simulink model "Delta"  (Simulink 7.7)
settings: Solver=ode45  StartTime=0.0  StopTime=40.0  RelTol=1e-3
undefined symbols (not defined in the file or in its folder): carriage, Printhead
libraries: mblibv1 x35
settings Model: Creator=Dot Com  LastModifiedBy=Dot Com
settings SimMechanicsCC: VisOnUpdateDiagram=on  VisDuringSimulation=on

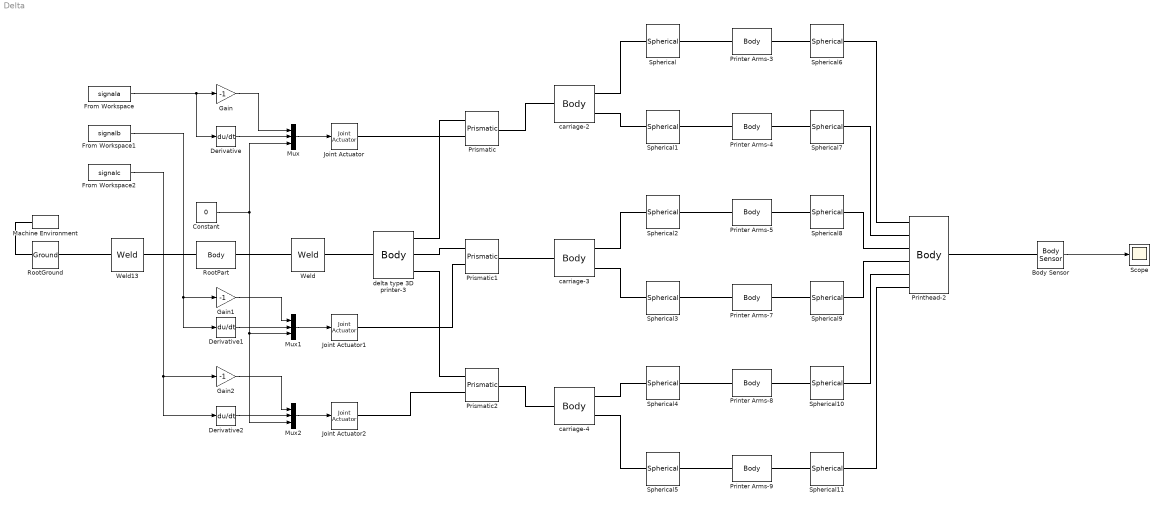
== system Delta ==
  Body Sensor : mblibv1/Sensors &  Actuators/Body Sensor  SystemSampleTime=-1  UpdateFromCAD=off  PhysicalDomain=Mechanical  PortType=blob  Muxed=on  Pose=off  Angle=on  AngleUnits=deg  ArcVelocity=off  ArcVelocityUnits=deg/s  ArcAcceleration=off  ArcAccelerationUnits=deg/s^2  CoordPosition=on  CoordPositionUnits=m  Velocity=off  VelocityUnits=m/s  Acceleration=off  AccelerationUnits=m/s^2  Quaternion=on  QuaternionDT=off  QuaternionDDT=off  QuaternionUnits=off  OutputVector=[1]  ActiveIO=on  Width=3  DialogClass=MechanicalSensorBlock  ReferenceFrame=Absolute (World)
  Constant : Constant  Value=0
  Derivative : Derivative
  Derivative1 : Derivative
  Derivative2 : Derivative
  From Workspace : FromWorkspace  VariableName=signala  SampleTime=0  OutputAfterFinalValue=Holding final value
  From Workspace1 : FromWorkspace  VariableName=signalb  SampleTime=0  OutputAfterFinalValue=Holding final value
  From Workspace2 : FromWorkspace  VariableName=signalc  SampleTime=0  OutputAfterFinalValue=Holding final value
  Gain : Gain  Gain=-1
  Gain1 : Gain  Gain=-1
  Gain2 : Gain  Gain=-1
  Joint Actuator : mblibv1/Sensors &  Actuators/Joint Actuator  SystemSampleTime=-1  UpdateFromCAD=off  PhysicalDomain=Mechanical  PortType=blob  ActuationStyle=Motion  AngleUnits=deg  ArcVelocityUnits=deg/s  ArcAccelerationUnits=deg/s^2  CoordPositionUnits=mm  VelocityUnits=mm/s  AccelerationUnits=mm/s^2  ForceUnits=N  TorqueUnits=N*m  ActiveIO=on  Width=3  DialogClass=MechanicalActuatorBlock  Primitive=P1  ReferenceFrame=Absolute (World)
  Joint Actuator1 : mblibv1/Sensors &  Actuators/Joint Actuator  SystemSampleTime=-1  UpdateFromCAD=off  PhysicalDomain=Mechanical  PortType=blob  ActuationStyle=Motion  AngleUnits=deg  ArcVelocityUnits=deg/s  ArcAccelerationUnits=deg/s^2  CoordPositionUnits=mm  VelocityUnits=mm/s  AccelerationUnits=mm/s^2  ForceUnits=N  TorqueUnits=N*m  ActiveIO=on  Width=3  DialogClass=MechanicalActuatorBlock  Primitive=P1  ReferenceFrame=Absolute (World)
  Joint Actuator2 : mblibv1/Sensors &  Actuators/Joint Actuator  SystemSampleTime=-1  UpdateFromCAD=off  PhysicalDomain=Mechanical  PortType=blob  ActuationStyle=Motion  AngleUnits=deg  ArcVelocityUnits=deg/s  ArcAccelerationUnits=deg/s^2  CoordPositionUnits=mm  VelocityUnits=mm/s  AccelerationUnits=mm/s^2  ForceUnits=N  TorqueUnits=N*m  ActiveIO=on  Width=3  DialogClass=MechanicalActuatorBlock  Primitive=P1  ReferenceFrame=Absolute (World)
  Machine Environment : mblibv1/Bodies/Machine Environment  SystemSampleTime=-1  PortType=env  PhysicalDomain=Mechanical  DialogTemplateClass=MECH.MachineEnvironment  SyncWhenCopied=off  Gravity=[0 -9.81 0]  GravityUnits=m/s^2  GravityAsSignal=off  Dimensionality=Auto-detect  AnalysisType=Forward dynamics  LinearAssemblyTolerance=1e-3  LinearAssemblyToleranceUnits=m  AngularAssemblyTolerance=1e-3  AngularAssemblyToleranceUnits=rad  ConstraintSolverType=Stabilizing  ConstraintRelTolerance=1e-4  ConstraintAbsTolerance=1e-4  UseRobustSingularityHandling=off  RedundancyAnalysisToleranceType=Automatically select tolerance  RedundancyAnalysisTolerance=1e-14  StatePerturbationType=Fixed  PerturbationSize=1e-5  VisualizeMachine=on  BodyVisualizationType=Use model default body geometries  BodyColorSelMode=Use model default  DefaultBodyColor=[1 0 0]
  Mux : Mux  Inputs=3
  Mux1 : Mux  Inputs=3
  Mux2 : Mux  Inputs=3
  Printer Arms-3 : mblibv1/Bodies/Body  PhysicalDomain=mechanical  SubClassName=Unknown  LeftPortType=workingframe  RightPortType=workingframe  LConnTagsString=CS2  RConnTagsString=CS3  UpdateFromCAD=on  PMImportedID=Printer Arms-3  DialogClass=MechanicalBodyBlock  Mass=0.000715383  MassUnits=kg  InertiaUnits=kg*m^2  Inertia=[6.53309e-006,-3.27611e-007,0;-3.27611e-007,1.87881e-008,0;0,0,6.55098e-006]  Shape=Cylinder  ShapeDims=[1 1]  ShapeUnits=m  ShapeUse=false  Density=1  DensityUnits=kg/m^3  DensityUse=false  GraphicsMode=GFXFILE  GraphicsFileName=Delta - Printer Arms-3.STL  BodyColorSelMode=COLORPALETTE  BodyColor=[0.752941;0.752941;0.752941]  AttachedToCS=CS1  CG=Right$CG$[-0.081798 0.287301 0.783358]$WORLD$WORLD$m$[0.856629 -0.438503 0.27185;0.422968 0.898604 0.11666;-0.295441 0.0150491 0.955242]$3x3 Transform$rad$WORLD$false$Printer Arms-3::CG(AUTOGEN)  WorkingFrames=Right$CS1$[0.0652951 0.305355 0.931629]$WORLD$WORLD$m$[0.856629 -0.438503 0.27185;0.422968 0.898604 0.11666;-0.295441 0.0150491 0.955242]$3x3 Transform$rad$WORLD$false$Printer Arms-3::CS1(AUTOGEN)#Left$CS2$[-0.126832 0.392029 0.78339]$WORLD$WORLD$m$[1 0 0;0 1 0;0 0 1]$3x3 Transform$rad$WORLD$true$Printer Arms-3:-:carriage-2::Printer Arms-3(AUTOGEN)#Right$CS3$[-0.0382516 0.186032 0.783333]$WORLD$WORLD$m$[1 0 0;0 1 0;0 0 1]$3x3 Transform$rad$WORLD$true$Printer Arms-3:-:Printhead-2::Printer Arms-3(AUTOGEN)  CGPos=[-0.081798 0.287301 0.783358]  CGRot=[0.856629 -0.438503 0.27185;0.422968 0.898604 0.11666;-0.295441 0.0150491 0.955242]  CS0Pos=[]  CS0Rot=[]  CS1Pos=[0.0652951 0.305355 0.931629]  CS1Rot=[0.856629 -0.438503 0.27185;0.422968 0.898604 0.11666;-0.295441 0.0150491 0.955242]  CS2Pos=[-0.126832 0.392029 0.78339]  CS2Rot=[1 0 0;0 1 0;0 0 1]  CS3Pos=[-0.0382516 0.186032 0.783333]  CS3Rot=[1 0 0;0 1 0;0 0 1]  CS4Pos=[]  CS4Rot=[]  CS5Pos=[]  CS5Rot=[]  CS6Pos=[]  CS6Rot=[]  CS7Pos=[]  CS7Rot=[]  CS8Pos=[]  CS8Rot=[]  CS9Pos=[]  CS9Rot=[]  CS10Pos=[]  CS10Rot=[]  CS11Pos=[]  CS11Rot=[]  CS12Pos=[]  CS12Rot=[]  CS13Pos=[]  CS13Rot=[]  CS14Pos=[]  CS14Rot=[]  CS15Pos=[]  CS15Rot=[]  CS16Pos=[]  CS16Rot=[]  CS17Pos=[]  CS17Rot=[]  CS18Pos=[]  CS18Rot=[]  CS19Pos=[]  CS19Rot=[]  CS20Pos=[]  CS20Rot=[]
  Printer Arms-4 : mblibv1/Bodies/Body  PhysicalDomain=mechanical  SubClassName=Unknown  LeftPortType=workingframe  RightPortType=workingframe  LConnTagsString=CS2  RConnTagsString=CS3  UpdateFromCAD=on  PMImportedID=Printer Arms-4  DialogClass=MechanicalBodyBlock  Mass=0.000715383  MassUnits=kg  InertiaUnits=kg*m^2  Inertia=[6.53309e-006,-3.27611e-007,0;-3.27611e-007,1.87881e-008,0;0,0,6.55098e-006]  Shape=Cylinder  ShapeDims=[1 1]  ShapeUnits=m  ShapeUse=false  Density=1  DensityUnits=kg/m^3  DensityUse=false  GraphicsMode=GFXFILE  GraphicsFileName=Delta - Printer Arms-4.STL  BodyColorSelMode=COLORPALETTE  BodyColor=[0.752941;0.752941;0.752941]  AttachedToCS=CS1  CG=Right$CG$[-0.081798 0.287301 0.744332]$WORLD$WORLD$m$[0.857774 -0.438561 0.268119;0.423387 0.898583 0.115293;-0.29149 0.0146226 0.956462]$3x3 Transform$rad$WORLD$false$Printer Arms-4::CG(AUTOGEN)  WorkingFrames=Right$CS1$[0.0647153 0.305142 0.893201]$WORLD$WORLD$m$[0.857774 -0.438561 0.268119;0.423387 0.898583 0.115293;-0.29149 0.0146226 0.956462]$3x3 Transform$rad$WORLD$false$Printer Arms-4::CS1(AUTOGEN)#Left$CS2$[-0.126832 0.392029 0.744338]$WORLD$WORLD$m$[1 0 0;0 1 0;0 0 1]$3x3 Transform$rad$WORLD$true$Printer Arms-4:-:carriage-2::Printer Arms-4(AUTOGEN)#Right$CS3$[-0.0382516 0.186032 0.744332]$WORLD$WORLD$m$[1 0 0;0 1 0;0 0 1]$3x3 Transform$rad$WORLD$true$Printer Arms-4:-:Printhead-2::Printer Arms-4(AUTOGEN)  CGPos=[-0.081798 0.287301 0.744332]  CGRot=[0.857774 -0.438561 0.268119;0.423387 0.898583 0.115293;-0.29149 0.0146226 0.956462]  CS0Pos=[]  CS0Rot=[]  CS1Pos=[0.0647153 0.305142 0.893201]  CS1Rot=[0.857774 -0.438561 0.268119;0.423387 0.898583 0.115293;-0.29149 0.0146226 0.956462]  CS2Pos=[-0.126832 0.392029 0.744338]  CS2Rot=[1 0 0;0 1 0;0 0 1]  CS3Pos=[-0.0382516 0.186032 0.744332]  CS3Rot=[1 0 0;0 1 0;0 0 1]  CS4Pos=[]  CS4Rot=[]  CS5Pos=[]  CS5Rot=[]  CS6Pos=[]  CS6Rot=[]  CS7Pos=[]  CS7Rot=[]  CS8Pos=[]  CS8Rot=[]  CS9Pos=[]  CS9Rot=[]  CS10Pos=[]  CS10Rot=[]  CS11Pos=[]  CS11Rot=[]  CS12Pos=[]  CS12Rot=[]  CS13Pos=[]  CS13Rot=[]  CS14Pos=[]  CS14Rot=[]  CS15Pos=[]  CS15Rot=[]  CS16Pos=[]  CS16Rot=[]  CS17Pos=[]  CS17Rot=[]  CS18Pos=[]  CS18Rot=[]  CS19Pos=[]  CS19Rot=[]  CS20Pos=[]  CS20Rot=[]
  Printer Arms-5 : mblibv1/Bodies/Body  PhysicalDomain=mechanical  SubClassName=Unknown  LeftPortType=workingframe  RightPortType=workingframe  LConnTagsString=CS2  RConnTagsString=CS3  UpdateFromCAD=on  PMImportedID=Printer Arms-5  DialogClass=MechanicalBodyBlock  Mass=0.000715383  MassUnits=kg  InertiaUnits=kg*m^2  Inertia=[6.53309e-006,-3.27611e-007,0;-3.27611e-007,1.87881e-008,0;0,0,6.55098e-006]  Shape=Cylinder  ShapeDims=[1 1]  ShapeUnits=m  ShapeUse=false  Density=1  DensityUnits=kg/m^3  DensityUse=false  GraphicsMode=GFXFILE  GraphicsFileName=Delta - Printer Arms-5.STL  BodyColorSelMode=COLORPALETTE  BodyColor=[0.752941;0.752941;0.752941]  AttachedToCS=CS1  CG=Right$CG$[0.0520521 0.287301 0.86061]$WORLD$WORLD$m$[0.619598 0.166684 -0.767017;-0.34181 0.936968 -0.0724985;0.706586 0.307094 0.637518]$3x3 Transform$rad$WORLD$false$Printer Arms-5::CG(AUTOGEN)  WorkingFrames=Right$CS1$[-0.0408836 0.200131 1.02708]$WORLD$WORLD$m$[0.619598 0.166684 -0.767017;-0.34181 0.936968 -0.0724985;0.706586 0.307094 0.637518]$3x3 Transform$rad$WORLD$false$Printer Arms-5::CS1(AUTOGEN)#Left$CS2$[0.0745745 0.392029 0.899608]$WORLD$WORLD$m$[1 0 0;0 1 0;0 0 1]$3x3 Transform$rad$WORLD$true$Printer Arms-5:-:carriage-3::Printer Arms-5(AUTOGEN)#Right$CS3$[0.0302789 0.186032 0.822898]$WORLD$WORLD$m$[1 0 0;0 1 0;0 0 1]$3x3 Transform$rad$WORLD$true$Printer Arms-5:-:Printhead-2::Printer Arms-5(AUTOGEN)  CGPos=[0.0520521 0.287301 0.86061]  CGRot=[0.619598 0.166684 -0.767017;-0.34181 0.936968 -0.0724985;0.706586 0.307094 0.637518]  CS0Pos=[]  CS0Rot=[]  CS1Pos=[-0.0408836 0.200131 1.02708]  CS1Rot=[0.619598 0.166684 -0.767017;-0.34181 0.936968 -0.0724985;0.706586 0.307094 0.637518]  CS2Pos=[0.0745745 0.392029 0.899608]  CS2Rot=[1 0 0;0 1 0;0 0 1]  CS3Pos=[0.0302789 0.186032 0.822898]  CS3Rot=[1 0 0;0 1 0;0 0 1]  CS4Pos=[]  CS4Rot=[]  CS5Pos=[]  CS5Rot=[]  CS6Pos=[]  CS6Rot=[]  CS7Pos=[]  CS7Rot=[]  CS8Pos=[]  CS8Rot=[]  CS9Pos=[]  CS9Rot=[]  CS10Pos=[]  CS10Rot=[]  CS11Pos=[]  CS11Rot=[]  CS12Pos=[]  CS12Rot=[]  CS13Pos=[]  CS13Rot=[]  CS14Pos=[]  CS14Rot=[]  CS15Pos=[]  CS15Rot=[]  CS16Pos=[]  CS16Rot=[]  CS17Pos=[]  CS17Rot=[]  CS18Pos=[]  CS18Rot=[]  CS19Pos=[]  CS19Rot=[]  CS20Pos=[]  CS20Rot=[]
  Printer Arms-7 : mblibv1/Bodies/Body  PhysicalDomain=mechanical  SubClassName=Unknown  LeftPortType=workingframe  RightPortType=workingframe  LConnTagsString=CS2  RConnTagsString=CS3  UpdateFromCAD=on  PMImportedID=Printer Arms-7  DialogClass=MechanicalBodyBlock  Mass=0.000715383  MassUnits=kg  InertiaUnits=kg*m^2  Inertia=[6.53309e-006,-3.27611e-007,0;-3.27611e-007,1.87881e-008,0;0,0,6.55098e-006]  Shape=Cylinder  ShapeDims=[1 1]  ShapeUnits=m  ShapeUse=false  Density=1  DensityUnits=kg/m^3  DensityUse=false  GraphicsMode=GFXFILE  GraphicsFileName=Delta - Printer Arms-7.STL  BodyColorSelMode=COLORPALETTE  BodyColor=[0.752941;0.752941;0.752941]  AttachedToCS=CS1  CG=Right$CG$[0.0858496 0.287301 0.841097]$WORLD$WORLD$m$[-0.593901 0.227756 0.771628;0.434444 0.898028 0.0693147;-0.677156 0.376395 -0.632287]$3x3 Transform$rad$WORLD$false$Printer Arms-7::CG(AUTOGEN)  WorkingFrames=Right$CS1$[0.163779 0.297714 0.646765]$WORLD$WORLD$m$[-0.593901 0.227756 0.771628;0.434444 0.898028 0.0693147;-0.677156 0.376395 -0.632287]$3x3 Transform$rad$WORLD$false$Printer Arms-7::CS1(AUTOGEN)#Left$CS2$[0.108395 0.392029 0.880082]$WORLD$WORLD$m$[1 0 0;0 1 0;0 0 1]$3x3 Transform$rad$WORLD$true$Printer Arms-7:-:carriage-3::Printer Arms-7(AUTOGEN)#Right$CS3$[0.0640546 0.186032 0.803398]$WORLD$WORLD$m$[1 0 0;0 1 0;0 0 1]$3x3 Transform$rad$WORLD$true$Printer Arms-7:-:Printhead-2::Printer Arms-7(AUTOGEN)  CGPos=[0.0858496 0.287301 0.841097]  CGRot=[-0.593901 0.227756 0.771628;0.434444 0.898028 0.0693147;-0.677156 0.376395 -0.632287]  CS0Pos=[]  CS0Rot=[]  CS1Pos=[0.163779 0.297714 0.646765]  CS1Rot=[-0.593901 0.227756 0.771628;0.434444 0.898028 0.0693147;-0.677156 0.376395 -0.632287]  CS2Pos=[0.108395 0.392029 0.880082]  CS2Rot=[1 0 0;0 1 0;0 0 1]  CS3Pos=[0.0640546 0.186032 0.803398]  CS3Rot=[1 0 0;0 1 0;0 0 1]  CS4Pos=[]  CS4Rot=[]  CS5Pos=[]  CS5Rot=[]  CS6Pos=[]  CS6Rot=[]  CS7Pos=[]  CS7Rot=[]  CS8Pos=[]  CS8Rot=[]  CS9Pos=[]  CS9Rot=[]  CS10Pos=[]  CS10Rot=[]  CS11Pos=[]  CS11Rot=[]  CS12Pos=[]  CS12Rot=[]  CS13Pos=[]  CS13Rot=[]  CS14Pos=[]  CS14Rot=[]  CS15Pos=[]  CS15Rot=[]  CS16Pos=[]  CS16Rot=[]  CS17Pos=[]  CS17Rot=[]  CS18Pos=[]  CS18Rot=[]  CS19Pos=[]  CS19Rot=[]  CS20Pos=[]  CS20Rot=[]
  Printer Arms-8 : mblibv1/Bodies/Body  PhysicalDomain=mechanical  SubClassName=Unknown  LeftPortType=workingframe  RightPortType=workingframe  LConnTagsString=CS2  RConnTagsString=CS3  UpdateFromCAD=on  PMImportedID=Printer Arms-8  DialogClass=MechanicalBodyBlock  Mass=0.000715383  MassUnits=kg  InertiaUnits=kg*m^2  Inertia=[6.53309e-006,-3.27611e-007,0;-3.27611e-007,1.87881e-008,0;0,0,6.55098e-006]  Shape=Cylinder  ShapeDims=[1 1]  ShapeUnits=m  ShapeUse=false  Density=1  DensityUnits=kg/m^3  DensityUse=false  GraphicsMode=GFXFILE  GraphicsFileName=Delta - Printer Arms-8.STL  BodyColorSelMode=COLORPALETTE  BodyColor=[0.752941;0.752941;0.752941]  AttachedToCS=CS1  CG=Right$CG$[0.0520296 0.287301 0.667041]$WORLD$WORLD$m$[-0.253842 0.210301 -0.944107;0.431532 0.898174 0.0840436;0.865647 -0.386079 -0.318746]$3x3 Transform$rad$WORLD$false$Printer Arms-8::CG(AUTOGEN)  WorkingFrames=Right$CS1$[-0.153917 0.300151 0.704021]$WORLD$WORLD$m$[-0.253842 0.210301 -0.944107;0.431532 0.898174 0.0840436;0.865647 -0.386079 -0.318746]$3x3 Transform$rad$WORLD$false$Printer Arms-8::CS1(AUTOGEN)#Left$CS2$[0.0745185 0.392029 0.628024]$WORLD$WORLD$m$[1 0 0;0 1 0;0 0 1]$3x3 Transform$rad$WORLD$true$Printer Arms-8:-:carriage-4::Printer Arms-8(AUTOGEN)#Right$CS3$[0.0302782 0.186032 0.704766]$WORLD$WORLD$m$[1 0 0;0 1 0;0 0 1]$3x3 Transform$rad$WORLD$true$Printer Arms-8:-:Printhead-2::Printer Arms-8(AUTOGEN)  CGPos=[0.0520296 0.287301 0.667041]  CGRot=[-0.253842 0.210301 -0.944107;0.431532 0.898174 0.0840436;0.865647 -0.386079 -0.318746]  CS0Pos=[]  CS0Rot=[]  CS1Pos=[-0.153917 0.300151 0.704021]  CS1Rot=[-0.253842 0.210301 -0.944107;0.431532 0.898174 0.0840436;0.865647 -0.386079 -0.318746]  CS2Pos=[0.0745185 0.392029 0.628024]  CS2Rot=[1 0 0;0 1 0;0 0 1]  CS3Pos=[0.0302782 0.186032 0.704766]  CS3Rot=[1 0 0;0 1 0;0 0 1]  CS4Pos=[]  CS4Rot=[]  CS5Pos=[]  CS5Rot=[]  CS6Pos=[]  CS6Rot=[]  CS7Pos=[]  CS7Rot=[]  CS8Pos=[]  CS8Rot=[]  CS9Pos=[]  CS9Rot=[]  CS10Pos=[]  CS10Rot=[]  CS11Pos=[]  CS11Rot=[]  CS12Pos=[]  CS12Rot=[]  CS13Pos=[]  CS13Rot=[]  CS14Pos=[]  CS14Rot=[]  CS15Pos=[]  CS15Rot=[]  CS16Pos=[]  CS16Rot=[]  CS17Pos=[]  CS17Rot=[]  CS18Pos=[]  CS18Rot=[]  CS19Pos=[]  CS19Rot=[]  CS20Pos=[]  CS20Rot=[]
  Printer Arms-9 : mblibv1/Bodies/Body  PhysicalDomain=mechanical  SubClassName=Unknown  LeftPortType=workingframe  RightPortType=workingframe  LConnTagsString=CS2  RConnTagsString=CS3  UpdateFromCAD=on  PMImportedID=Printer Arms-9  DialogClass=MechanicalBodyBlock  Mass=0.000715383  MassUnits=kg  InertiaUnits=kg*m^2  Inertia=[6.53309e-006,-3.27611e-007,0;-3.27611e-007,1.87881e-008,0;0,0,6.55098e-006]  Shape=Cylinder  ShapeDims=[1 1]  ShapeUnits=m  ShapeUse=false  Density=1  DensityUnits=kg/m^3  DensityUse=false  GraphicsMode=GFXFILE  GraphicsFileName=Delta - Printer Arms-9.STL  BodyColorSelMode=COLORPALETTE  BodyColor=[0.752941;0.752941;0.752941]  AttachedToCS=CS1  CG=Right$CG$[0.0858271 0.287301 0.686554]$WORLD$WORLD$m$[-0.257215 0.210668 -0.943111;0.431786 0.898161 0.0828664;0.864524 -0.385908 -0.321984]$3x3 Transform$rad$WORLD$false$Printer Arms-9::CG(AUTOGEN)  WorkingFrames=Right$CS1$[-0.120256 0.299959 0.72283]$WORLD$WORLD$m$[-0.257215 0.210668 -0.943111;0.431786 0.898161 0.0828664;0.864524 -0.385908 -0.321984]$3x3 Transform$rad$WORLD$false$Printer Arms-9::CS1(AUTOGEN)#Left$CS2$[0.108339 0.392029 0.64755]$WORLD$WORLD$m$[1 0 0;0 1 0;0 0 1]$3x3 Transform$rad$WORLD$true$Printer Arms-9:-:carriage-4::Printer Arms-9(AUTOGEN)#Right$CS3$[0.0640539 0.186032 0.724266]$WORLD$WORLD$m$[1 0 0;0 1 0;0 0 1]$3x3 Transform$rad$WORLD$true$Printer Arms-9:-:Printhead-2::Printer Arms-9(AUTOGEN)  CGPos=[0.0858271 0.287301 0.686554]  CGRot=[-0.257215 0.210668 -0.943111;0.431786 0.898161 0.0828664;0.864524 -0.385908 -0.321984]  CS0Pos=[]  CS0Rot=[]  CS1Pos=[-0.120256 0.299959 0.72283]  CS1Rot=[-0.257215 0.210668 -0.943111;0.431786 0.898161 0.0828664;0.864524 -0.385908 -0.321984]  CS2Pos=[0.108339 0.392029 0.64755]  CS2Rot=[1 0 0;0 1 0;0 0 1]  CS3Pos=[0.0640539 0.186032 0.724266]  CS3Rot=[1 0 0;0 1 0;0 0 1]  CS4Pos=[]  CS4Rot=[]  CS5Pos=[]  CS5Rot=[]  CS6Pos=[]  CS6Rot=[]  CS7Pos=[]  CS7Rot=[]  CS8Pos=[]  CS8Rot=[]  CS9Pos=[]  CS9Rot=[]  CS10Pos=[]  CS10Rot=[]  CS11Pos=[]  CS11Rot=[]  CS12Pos=[]  CS12Rot=[]  CS13Pos=[]  CS13Rot=[]  CS14Pos=[]  CS14Rot=[]  CS15Pos=[]  CS15Rot=[]  CS16Pos=[]  CS16Rot=[]  CS17Pos=[]  CS17Rot=[]  CS18Pos=[]  CS18Rot=[]  CS19Pos=[]  CS19Rot=[]  CS20Pos=[]  CS20Rot=[]
  Printhead-2 : mblibv1/Bodies/Body  PhysicalDomain=mechanical  SubClassName=Unknown  LeftPortType=workingframe  RightPortType=workingframe  LConnTagsString=CS2|CS3|CS4|CS5|CS6|CS7  RConnTagsString=CS1  UpdateFromCAD=on  PMImportedID=Printhead-2  DialogClass=MechanicalBodyBlock  Mass=0.132596  MassUnits=kg  InertiaUnits=kg*m^2  Inertia=[0.000117863,0,0;0,0.000230731,0;0,0,0.000117863]  Shape=Cylinder  ShapeDims=[1 1]  ShapeUnits=m  ShapeUse=false  Density=1  DensityUnits=kg/m^3  DensityUse=false  GraphicsMode=GFXFILE  GraphicsFileName=Delta - Printhead-2.STL  BodyColorSelMode=COLORPALETTE  BodyColor=[0.75294 0.75294 0.75294]  AttachedToCS=CS1  CG=Right$CG$[0.0186937 0.182574 0.763832]$WORLD$WORLD$m$[-3.8521e-007 0 -1;-1.23652e-012 1 0;1 1.23652e-012 -3.8521e-007]$3x3 Transform$rad$WORLD$false$Printhead-2::CG(AUTOGEN)  WorkingFrames=Right$CS1$[0.146711 0.19172 0.763551]$WORLD$WORLD$m$[-3.8521e-007 0 -1;-1.23652e-012 1 0;1 1.23652e-012 -3.8521e-007]$3x3 Transform$rad$WORLD$true$Printhead-2::CS1(AUTOGEN)#Left$CS2$[-0.0382516 0.186032 0.783333]$WORLD$WORLD$m$[1 0 0;0 1 0;0 0 1]$3x3 Transform$rad$WORLD$true$Printer Arms-3:-:Printhead-2::Printhead-2(AUTOGEN)#Left$CS3$[-0.0382516 0.186032 0.744332]$WORLD$WORLD$m$[1 0 0;0 1 0;0 0 1]$3x3 Transform$rad$WORLD$true$Printer Arms-4:-:Printhead-2::Printhead-2(AUTOGEN)#Left$CS4$[0.0302789 0.186032 0.822898]$WORLD$WORLD$m$[1 0 0;0 1 0;0 0 1]$3x3 Transform$rad$WORLD$true$Printer Arms-5:-:Printhead-2::Printhead-2(AUTOGEN)#Left$CS5$[0.0640546 0.186032 0.803398]$WORLD$WORLD$m$[1 0 0;0 1 0;0 0 1]$3x3 Transform$rad$WORLD$true$Printer Arms-7:-:Printhead-2::Printhead-2(AUTOGEN)#Left$CS6$[0.0302782 0.186032 0.704766]$WORLD$WORLD$m$[1 0 0;0 1 0;0 0 1]$3x3 Transform$rad$WORLD$true$Printer Arms-8:-:Printhead-2::Printhead-2(AUTOGEN)#Left$CS7$[0.0640539 0.186032 0.724266]$WORLD$WORLD$m$[1 0 0;0 1 0;0 0 1]$3x3 Transform$rad$WORLD$true$Printer Arms-9:-:Printhead-2::Printhead-2(AUTOGEN)  CGPos=[0.0186937 0.182574 0.763832]  CGRot=[-3.8521e-007 0 -1;-1.23652e-012 1 0;1 1.23652e-012 -3.8521e-007]  CS0Pos=[]  CS0Rot=[]  CS1Pos=[0.146711 0.19172 0.763551]  CS1Rot=[-3.8521e-007 0 -1;-1.23652e-012 1 0;1 1.23652e-012 -3.8521e-007]  CS2Pos=[-0.0382516 0.186032 0.783333]  CS2Rot=[1 0 0;0 1 0;0 0 1]  CS3Pos=[-0.0382516 0.186032 0.744332]  CS3Rot=[1 0 0;0 1 0;0 0 1]  CS4Pos=[0.0302789 0.186032 0.822898]  CS4Rot=[1 0 0;0 1 0;0 0 1]  CS5Pos=[0.0640546 0.186032 0.803398]  CS5Rot=[1 0 0;0 1 0;0 0 1]  CS6Pos=[0.0302782 0.186032 0.704766]  CS6Rot=[1 0 0;0 1 0;0 0 1]  CS7Pos=[0.0640539 0.186032 0.724266]  CS7Rot=[1 0 0;0 1 0;0 0 1]  CS8Pos=[]  CS8Rot=[]  CS9Pos=[]  CS9Rot=[]  CS10Pos=[]  CS10Rot=[]  CS11Pos=[]  CS11Rot=[]  CS12Pos=[]  CS12Rot=[]  CS13Pos=[]  CS13Rot=[]  CS14Pos=[]  CS14Rot=[]  CS15Pos=[]  CS15Rot=[]  CS16Pos=[]  CS16Rot=[]  CS17Pos=[]  CS17Rot=[]  CS18Pos=[]  CS18Rot=[]  CS19Pos=[]  CS19Rot=[]  CS20Pos=[]  CS20Rot=[]
  Prismatic : mblibv1/Joints/Prismatic  PhysicalDomain=mechanical  SubClassName=Unknown  LeftPortType=blob  RightPortType=blob  LConnTagsString=__newl0|SA1  RConnTagsString=__newr0  UpdateFromCAD=on  PMImportedID=carriage-2:-:delta type 3D printer-3  NumSAPorts=1  CutJoint=off  MarkAsCut=off  Primitives=prismatic  PrimitiveProps=P1$World$[0,1,0]$prismatic  DialogClass=JointBlock  P1Axis=[0,1,0]
  Prismatic1 : mblibv1/Joints/Prismatic  PhysicalDomain=mechanical  SubClassName=Unknown  LeftPortType=blob  RightPortType=blob  LConnTagsString=__newl0|SA1  RConnTagsString=__newr0  UpdateFromCAD=on  PMImportedID=carriage-3:-:delta type 3D printer-3  NumSAPorts=1  CutJoint=off  MarkAsCut=off  Primitives=prismatic  PrimitiveProps=P1$World$[0,1,0]$prismatic  DialogClass=JointBlock  P1Axis=[0,1,0]
  Prismatic2 : mblibv1/Joints/Prismatic  PhysicalDomain=mechanical  SubClassName=Unknown  LeftPortType=blob  RightPortType=blob  LConnTagsString=__newl0|SA1  RConnTagsString=__newr0  UpdateFromCAD=on  PMImportedID=carriage-4:-:delta type 3D printer-3  NumSAPorts=1  CutJoint=off  MarkAsCut=off  Primitives=prismatic  PrimitiveProps=P1$World$[0,1,0]$prismatic  DialogClass=JointBlock  P1Axis=[0,1,0]
  RootGround : mblibv1/Bodies/Ground  SystemSampleTime=-1  UpdateFromCAD=on  PMImportedID=RootGround  LeftPortType=env  RightPortType=workingframe  PhysicalDomain=Mechanical  DialogClass=GroundBlock  CoordPosition=[0.0186634,0.0298068,0.763791]  CoordPositionUnits=m  StateVectorMgrId=1  MachineId=[2 0]  ShowEnvPort=on
  RootPart : mblibv1/Bodies/Body  PhysicalDomain=mechanical  SubClassName=Unknown  LeftPortType=workingframe  RightPortType=workingframe  LConnTagsString=CS3  RConnTagsString=CS2  UpdateFromCAD=on  PMImportedID=Delta/RootPart  DialogClass=MechanicalBodyBlock  Mass=0  MassUnits=kg  InertiaUnits=kg*m^2  Inertia=[0,0,0;0,0,0;0,0,0]  Shape=Cylinder  ShapeDims=[1 1]  ShapeUnits=m  ShapeUse=false  Density=1  DensityUnits=kg/m^3  DensityUse=false  GraphicsMode=MACHINE_DEFAULT  BodyColorSelMode=MACHINE_DEFAULT  BodyColor=[1;0;0]  AttachedToCS=CS1  CG=Right$CG$[0.0186634 0.0298068 0.763791]$WORLD$WORLD$m$[1 0 0;0 1 0;0 0 1]$3x3 Transform$rad$WORLD$false$Delta/RootPart::CG(AUTOGEN)  WorkingFrames=Right$CS1$[0 0 0]$WORLD$WORLD$m$[1 0 0;0 1 0;0 0 1]$3x3 Transform$rad$WORLD$false$Delta/RootPart::CS1(AUTOGEN)#Right$CS2$[0.0186587 -0.0166149 0.763785]$WORLD$WORLD$m$[1 0 0;0 1 0;0 0 1]$3x3 Transform$rad$WORLD$true$Delta/RootPart:-:delta type 3D printer-3::Delta/RootPart(AUTOGEN)#Left$CS3$[0.0186634 0.0298068 0.763791]$WORLD$WORLD$m$[1 0 0;0 1 0;0 0 1]$3x3 Transform$rad$WORLD$true$Delta/RootPart:-:RootGround::Delta/RootPart(AUTOGEN)  CGPos=[0.0186634 0.0298068 0.763791]  CGRot=[1 0 0;0 1 0;0 0 1]  CS0Pos=[]  CS0Rot=[]  CS1Pos=[0 0 0]  CS1Rot=[1 0 0;0 1 0;0 0 1]  CS2Pos=[0.0186587 -0.0166149 0.763785]  CS2Rot=[1 0 0;0 1 0;0 0 1]  CS3Pos=[0.0186634 0.0298068 0.763791]  CS3Rot=[1 0 0;0 1 0;0 0 1]  CS4Pos=[]  CS4Rot=[]  CS5Pos=[]  CS5Rot=[]  CS6Pos=[]  CS6Rot=[]  CS7Pos=[]  CS7Rot=[]  CS8Pos=[]  CS8Rot=[]  CS9Pos=[]  CS9Rot=[]  CS10Pos=[]  CS10Rot=[]  CS11Pos=[]  CS11Rot=[]  CS12Pos=[]  CS12Rot=[]  CS13Pos=[]  CS13Rot=[]  CS14Pos=[]  CS14Rot=[]  CS15Pos=[]  CS15Rot=[]  CS16Pos=[]  CS16Rot=[]  CS17Pos=[]  CS17Rot=[]  CS18Pos=[]  CS18Rot=[]  CS19Pos=[]  CS19Rot=[]  CS20Pos=[]  CS20Rot=[]
  Scope : Scope
  Spherical{,1..11} (12 alike) : mblibv1/Joints/Spherical  PhysicalDomain=mechanical  SubClassName=Unknown  LeftPortType=blob  RightPortType=blob  LConnTagsString=__newl0  RConnTagsString=__newr0  UpdateFromCAD=off  NumSAPorts=0  CutJoint=off  MarkAsCut=off  Primitives=spherical  PrimitiveProps=S$WORLD$[0 0 0]$spherical  DialogClass=JointBlock  SAxis=[0 0 0]
  Weld : mblibv1/Joints/Weld  PhysicalDomain=mechanical  SubClassName=Unknown  LeftPortType=blob  RightPortType=blob  LConnTagsString=__newl0  RConnTagsString=__newr0  UpdateFromCAD=on  PMImportedID=Delta/RootPart:-:delta type 3D printer-3  NumSAPorts=0  CutJoint=off  MarkAsCut=off  Primitives=weld  PrimitiveProps=W$WORLD$[0.57735,0.57735,0.57735]$weld  DialogClass=JointBlock  WAxis=[0.57735,0.57735,0.57735]
  Weld13 : mblibv1/Joints/Weld  PhysicalDomain=mechanical  SubClassName=Unknown  LeftPortType=blob  RightPortType=blob  LConnTagsString=__newl0  RConnTagsString=__newr0  UpdateFromCAD=on  PMImportedID=Delta/RootPart:-:RootGround  NumSAPorts=0  CutJoint=off  MarkAsCut=off  Primitives=weld  PrimitiveProps=W$WORLD$[0.57735,0.57735,0.57735]$weld  DialogClass=JointBlock  WAxis=[0.57735,0.57735,0.57735]
  carriage-2 : mblibv1/Bodies/Body  PhysicalDomain=mechanical  SubClassName=Unknown  LeftPortType=workingframe  RightPortType=workingframe  LConnTagsString=CS2  RConnTagsString=CS3|CS4  UpdateFromCAD=on  PMImportedID=carriage-2  DialogClass=MechanicalBodyBlock  Mass=0.119531  MassUnits=kg  InertiaUnits=kg*m^2  Inertia=[8.71516e-005,1.3952e-008,-7.11667e-010;1.3952e-008,0.000105618,4.08463e-013;-7.11667e-010,4.08463e-013,5.02939e-005]  Shape=Cylinder  ShapeDims=[1 1]  ShapeUnits=m  ShapeUse=false  Density=1  DensityUnits=kg/m^3  DensityUse=false  GraphicsMode=GFXFILE  GraphicsFileName=Delta - carriage-2.STL  BodyColorSelMode=COLORPALETTE  BodyColor=[0.752941;0.752941;0.752941]  AttachedToCS=CS1  CG=Right$CG$[-0.146483 0.392017 0.763832]$WORLD$WORLD$m$[-1 0 0;0 1 0;0 0 -1]$3x3 Transform$rad$WORLD$false$carriage-2::CG(AUTOGEN)  WorkingFrames=Right$CS1$[-0.157413 0.388666 0.853832]$WORLD$WORLD$m$[-1 0 0;0 1 0;0 0 -1]$3x3 Transform$rad$WORLD$false$carriage-2::CS1(AUTOGEN)#Left$CS2$[-0.156832 0.412029 0.733832]$WORLD$WORLD$m$[1 0 0;0 1 0;0 0 1]$3x3 Transform$rad$WORLD$true$carriage-2:-:delta type 3D printer-3::carriage-2(AUTOGEN)#Right$CS3$[-0.126832 0.392029 0.78339]$WORLD$WORLD$m$[1 0 0;0 1 0;0 0 1]$3x3 Transform$rad$WORLD$true$Printer Arms-3:-:carriage-2::carriage-2(AUTOGEN)#Right$CS4$[-0.126832 0.392029 0.744338]$WORLD$WORLD$m$[1 0 0;0 1 0;0 0 1]$3x3 Transform$rad$WORLD$true$Printer Arms-4:-:carriage-2::carriage-2(AUTOGEN)  CGPos=[-0.146483 0.392017 0.763832]  CGRot=[-1 0 0;0 1 0;0 0 -1]  CS0Pos=[]  CS0Rot=[]  CS1Pos=[-0.157413 0.388666 0.853832]  CS1Rot=[-1 0 0;0 1 0;0 0 -1]  CS2Pos=[-0.156832 0.412029 0.733832]  CS2Rot=[1 0 0;0 1 0;0 0 1]  CS3Pos=[-0.126832 0.392029 0.78339]  CS3Rot=[1 0 0;0 1 0;0 0 1]  CS4Pos=[-0.126832 0.392029 0.744338]  CS4Rot=[1 0 0;0 1 0;0 0 1]  CS5Pos=[]  CS5Rot=[]  CS6Pos=[]  CS6Rot=[]  CS7Pos=[]  CS7Rot=[]  CS8Pos=[]  CS8Rot=[]  CS9Pos=[]  CS9Rot=[]  CS10Pos=[]  CS10Rot=[]  CS11Pos=[]  CS11Rot=[]  CS12Pos=[]  CS12Rot=[]  CS13Pos=[]  CS13Rot=[]  CS14Pos=[]  CS14Rot=[]  CS15Pos=[]  CS15Rot=[]  CS16Pos=[]  CS16Rot=[]  CS17Pos=[]  CS17Rot=[]  CS18Pos=[]  CS18Rot=[]  CS19Pos=[]  CS19Rot=[]  CS20Pos=[]  CS20Rot=[]
  carriage-3 : mblibv1/Bodies/Body  PhysicalDomain=mechanical  SubClassName=Unknown  LeftPortType=workingframe  RightPortType=workingframe  LConnTagsString=CS2  RConnTagsString=CS3|CS4  UpdateFromCAD=on  PMImportedID=carriage-3  DialogClass=MechanicalBodyBlock  Mass=0.119531  MassUnits=kg  InertiaUnits=kg*m^2  Inertia=[8.71516e-005,1.3952e-008,-7.11667e-010;1.3952e-008,0.000105618,4.08463e-013;-7.11667e-010,4.08463e-013,5.02939e-005]  Shape=Cylinder  ShapeDims=[1 1]  ShapeUnits=m  ShapeUse=false  Density=1  DensityUnits=kg/m^3  DensityUse=false  GraphicsMode=GFXFILE  GraphicsFileName=Delta - carriage-3.STL  BodyColorSelMode=COLORPALETTE  BodyColor=[0.752941;0.752941;0.752941]  AttachedToCS=CS1  CG=Right$CG$[0.101282 0.392017 0.906879]$WORLD$WORLD$m$[0.5 0 -0.866025;0 1 0;0.866025 0 0.5]$3x3 Transform$rad$WORLD$false$carriage-3::CG(AUTOGEN)  WorkingFrames=Right$CS1$[0.184689 0.388666 0.871345]$WORLD$WORLD$m$[0.5 0 -0.866025;0 1 0;0.866025 0 0.5]$3x3 Transform$rad$WORLD$false$carriage-3::CS1(AUTOGEN)#Left$CS2$[0.0804758 0.412029 0.930842]$WORLD$WORLD$m$[1 0 0;0 1 0;0 0 1]$3x3 Transform$rad$WORLD$true$carriage-3:-:delta type 3D printer-3::carriage-3(AUTOGEN)#Right$CS3$[0.0745745 0.392029 0.899608]$WORLD$WORLD$m$[1 0 0;0 1 0;0 0 1]$3x3 Transform$rad$WORLD$true$Printer Arms-5:-:carriage-3::carriage-3(AUTOGEN)#Right$CS4$[0.108395 0.392029 0.880082]$WORLD$WORLD$m$[1 0 0;0 1 0;0 0 1]$3x3 Transform$rad$WORLD$true$Printer Arms-7:-:carriage-3::carriage-3(AUTOGEN)  CGPos=[0.101282 0.392017 0.906879]  CGRot=[0.5 0 -0.866025;0 1 0;0.866025 0 0.5]  CS0Pos=[]  CS0Rot=[]  CS1Pos=[0.184689 0.388666 0.871345]  CS1Rot=[0.5 0 -0.866025;0 1 0;0.866025 0 0.5]  CS2Pos=[0.0804758 0.412029 0.930842]  CS2Rot=[1 0 0;0 1 0;0 0 1]  CS3Pos=[0.0745745 0.392029 0.899608]  CS3Rot=[1 0 0;0 1 0;0 0 1]  CS4Pos=[0.108395 0.392029 0.880082]  CS4Rot=[1 0 0;0 1 0;0 0 1]  CS5Pos=[]  CS5Rot=[]  CS6Pos=[]  CS6Rot=[]  CS7Pos=[]  CS7Rot=[]  CS8Pos=[]  CS8Rot=[]  CS9Pos=[]  CS9Rot=[]  CS10Pos=[]  CS10Rot=[]  CS11Pos=[]  CS11Rot=[]  CS12Pos=[]  CS12Rot=[]  CS13Pos=[]  CS13Rot=[]  CS14Pos=[]  CS14Rot=[]  CS15Pos=[]  CS15Rot=[]  CS16Pos=[]  CS16Rot=[]  CS17Pos=[]  CS17Rot=[]  CS18Pos=[]  CS18Rot=[]  CS19Pos=[]  CS19Rot=[]  CS20Pos=[]  CS20Rot=[]
  carriage-4 : mblibv1/Bodies/Body  PhysicalDomain=mechanical  SubClassName=Unknown  LeftPortType=workingframe  RightPortType=workingframe  LConnTagsString=CS2  RConnTagsString=CS3|CS4  UpdateFromCAD=on  PMImportedID=carriage-4  DialogClass=MechanicalBodyBlock  Mass=0.119531  MassUnits=kg  InertiaUnits=kg*m^2  Inertia=[8.71516e-005,1.3952e-008,-7.11667e-010;1.3952e-008,0.000105618,4.08463e-013;-7.11667e-010,4.08463e-013,5.02939e-005]  Shape=Cylinder  ShapeDims=[1 1]  ShapeUnits=m  ShapeUse=false  Density=1  DensityUnits=kg/m^3  DensityUse=false  GraphicsMode=GFXFILE  GraphicsFileName=Delta - carriage-4.STL  BodyColorSelMode=COLORPALETTE  BodyColor=[0.752941;0.752941;0.752941]  AttachedToCS=CS1  CG=Right$CG$[0.101282 0.392017 0.620785]$WORLD$WORLD$m$[0.5 0 0.866025;0 1 0;-0.866025 0 0.5]$3x3 Transform$rad$WORLD$false$carriage-4::CG(AUTOGEN)  WorkingFrames=Right$CS1$[0.0288049 0.388666 0.566319]$WORLD$WORLD$m$[0.5 0 0.866025;0 1 0;-0.866025 0 0.5]$3x3 Transform$rad$WORLD$false$carriage-4::CS1(AUTOGEN)#Left$CS2$[0.0804758 0.412029 0.596822]$WORLD$WORLD$m$[1 0 0;0 1 0;0 0 1]$3x3 Transform$rad$WORLD$true$carriage-4:-:delta type 3D printer-3::carriage-4(AUTOGEN)#Right$CS3$[0.0745185 0.392029 0.628024]$WORLD$WORLD$m$[1 0 0;0 1 0;0 0 1]$3x3 Transform$rad$WORLD$true$Printer Arms-8:-:carriage-4::carriage-4(AUTOGEN)#Right$CS4$[0.108339 0.392029 0.64755]$WORLD$WORLD$m$[1 0 0;0 1 0;0 0 1]$3x3 Transform$rad$WORLD$true$Printer Arms-9:-:carriage-4::carriage-4(AUTOGEN)  CGPos=[0.101282 0.392017 0.620785]  CGRot=[0.5 0 0.866025;0 1 0;-0.866025 0 0.5]  CS0Pos=[]  CS0Rot=[]  CS1Pos=[0.0288049 0.388666 0.566319]  CS1Rot=[0.5 0 0.866025;0 1 0;-0.866025 0 0.5]  CS2Pos=[0.0804758 0.412029 0.596822]  CS2Rot=[1 0 0;0 1 0;0 0 1]  CS3Pos=[0.0745185 0.392029 0.628024]  CS3Rot=[1 0 0;0 1 0;0 0 1]  CS4Pos=[0.108339 0.392029 0.64755]  CS4Rot=[1 0 0;0 1 0;0 0 1]  CS5Pos=[]  CS5Rot=[]  CS6Pos=[]  CS6Rot=[]  CS7Pos=[]  CS7Rot=[]  CS8Pos=[]  CS8Rot=[]  CS9Pos=[]  CS9Rot=[]  CS10Pos=[]  CS10Rot=[]  CS11Pos=[]  CS11Rot=[]  CS12Pos=[]  CS12Rot=[]  CS13Pos=[]  CS13Rot=[]  CS14Pos=[]  CS14Rot=[]  CS15Pos=[]  CS15Rot=[]  CS16Pos=[]  CS16Rot=[]  CS17Pos=[]  CS17Rot=[]  CS18Pos=[]  CS18Rot=[]  CS19Pos=[]  CS19Rot=[]  CS20Pos=[]  CS20Rot=[]
  delta type 3D printer-3 : mblibv1/Bodies/Body  PhysicalDomain=mechanical  SubClassName=Unknown  LeftPortType=workingframe  RightPortType=workingframe  LConnTagsString=CS2  RConnTagsString=CS3|CS4|CS5  UpdateFromCAD=on  PMImportedID=delta type 3D printer-3  DialogClass=MechanicalBodyBlock  Mass=3.25813  MassUnits=kg  InertiaUnits=kg*m^2  Inertia=[0.36389,-2.65999e-006,3.41661e-005;-2.65999e-006,0.36387,2.64566e-005;3.41661e-005,2.64566e-005,0.0593532]  Shape=Cylinder  ShapeDims=[1 1]  ShapeUnits=m  ShapeUse=false  Density=1  DensityUnits=kg/m^3  DensityUse=false  GraphicsMode=GFXFILE  GraphicsFileName=Delta - delta type 3D printer-3.STL  BodyColorSelMode=COLORPALETTE  BodyColor=[0.752941;0.752941;0.752941]  AttachedToCS=CS1  CG=Right$CG$[0.0186587 -0.0166149 0.763785]$WORLD$WORLD$m$[0 -1 0;0 0 1;-1 0 0]$3x3 Transform$rad$WORLD$false$delta type 3D printer-3::CG(AUTOGEN)  WorkingFrames=Right$CS1$[0.234956 -0.535705 0.915441]$WORLD$WORLD$m$[0 -1 0;0 0 1;-1 0 0]$3x3 Transform$rad$WORLD$false$delta type 3D printer-3::CS1(AUTOGEN)#Left$CS2$[0.0186587 -0.0166149 0.763785]$WORLD$WORLD$m$[1 0 0;0 1 0;0 0 1]$3x3 Transform$rad$WORLD$true$Delta/RootPart:-:delta type 3D printer-3::delta type 3D printer-3(AUTOGEN)#Right$CS3$[-0.156832 0.442029 0.733832]$WORLD$WORLD$m$[1 0 0;0 1 0;0 0 1]$3x3 Transform$rad$WORLD$true$carriage-2:-:delta type 3D printer-3::delta type 3D printer-3(AUTOGEN)#Right$CS4$[0.0804758 0.442029 0.930842]$WORLD$WORLD$m$[1 0 0;0 1 0;0 0 1]$3x3 Transform$rad$WORLD$true$carriage-3:-:delta type 3D printer-3::delta type 3D printer-3(AUTOGEN)#Right$CS5$[0.0804758 0.442029 0.596822]$WORLD$WORLD$m$[1 0 0;0 1 0;0 0 1]$3x3 Transform$rad$WORLD$true$carriage-4:-:delta type 3D printer-3::delta type 3D printer-3(AUTOGEN)  CGPos=[0.0186587 -0.0166149 0.763785]  CGRot=[0 -1 0;0 0 1;-1 0 0]  CS0Pos=[]  CS0Rot=[]  CS1Pos=[0.234956 -0.535705 0.915441]  CS1Rot=[0 -1 0;0 0 1;-1 0 0]  CS2Pos=[0.0186587 -0.0166149 0.763785]  CS2Rot=[1 0 0;0 1 0;0 0 1]  CS3Pos=[-0.156832 0.442029 0.733832]  CS3Rot=[1 0 0;0 1 0;0 0 1]  CS4Pos=[0.0804758 0.442029 0.930842]  CS4Rot=[1 0 0;0 1 0;0 0 1]  CS5Pos=[0.0804758 0.442029 0.596822]  CS5Rot=[1 0 0;0 1 0;0 0 1]  CS6Pos=[]  CS6Rot=[]  CS7Pos=[]  CS7Rot=[]  CS8Pos=[]  CS8Rot=[]  CS9Pos=[]  CS9Rot=[]  CS10Pos=[]  CS10Rot=[]  CS11Pos=[]  CS11Rot=[]  CS12Pos=[]  CS12Rot=[]  CS13Pos=[]  CS13Rot=[]  CS14Pos=[]  CS14Rot=[]  CS15Pos=[]  CS15Rot=[]  CS16Pos=[]  CS16Rot=[]  CS17Pos=[]  CS17Rot=[]  CS18Pos=[]  CS18Rot=[]  CS19Pos=[]  CS19Rot=[]  CS20Pos=[]  CS20Rot=[]
  wires:
  Mux/1 -> Joint Actuator/1
  Mux1/1 -> Joint Actuator1/1
  Mux2/1 -> Joint Actuator2/1
  Derivative2/1 -> Mux2/2
  Derivative1/1 -> Mux1/2
  Derivative/1 -> Mux/2
  Constant/1 -> Mux/3, Mux1/3, Mux2/3
  Gain2/1 -> Mux2/1
  Gain1/1 -> Mux1/1
  Gain/1 -> Mux/1
  From Workspace/1 -> Gain/1, Derivative/1
  From Workspace1/1 -> Gain1/1, Derivative1/1
  From Workspace2/1 -> Gain2/1, Derivative2/1
  Body Sensor/1 -> Scope/1
  connections:
  RootPart/RConn1 -- Weld/LConn1
  Weld/RConn1 -- delta type 3D printer-3/LConn1
  delta type 3D printer-3/RConn1 -- Prismatic/LConn1
  Prismatic/RConn1 -- carriage-2/LConn1
  delta type 3D printer-3/RConn2 -- Prismatic1/LConn1
  Prismatic1/RConn1 -- carriage-3/LConn1
  delta type 3D printer-3/RConn3 -- Prismatic2/LConn1
  Prismatic2/RConn1 -- carriage-4/LConn1
  carriage-2/RConn1 -- Spherical/LConn1
  Spherical/RConn1 -- Printer Arms-3/LConn1
  carriage-2/RConn2 -- Spherical1/LConn1
  Spherical1/RConn1 -- Printer Arms-4/LConn1
  carriage-3/RConn1 -- Spherical2/LConn1
  Spherical2/RConn1 -- Printer Arms-5/LConn1
  carriage-3/RConn2 -- Spherical3/LConn1
  Spherical3/RConn1 -- Printer Arms-7/LConn1
  carriage-4/RConn1 -- Spherical4/LConn1
  Spherical4/RConn1 -- Printer Arms-8/LConn1
  RootGround/RConn1 -- Weld13/LConn1
  Weld13/RConn1 -- RootPart/LConn1
  RootGround/LConn1 -- Machine Environment/RConn1
  Joint Actuator/RConn1 -- Prismatic/LConn2
  Joint Actuator1/RConn1 -- Prismatic1/LConn2
  Joint Actuator2/RConn1 -- Prismatic2/LConn2
  carriage-4/RConn2 -- Spherical5/LConn1
  Spherical5/RConn1 -- Printer Arms-9/LConn1
  Printer Arms-9/RConn1 -- Spherical11/LConn1
  Spherical11/RConn1 -- Printhead-2/LConn6
  Spherical10/RConn1 -- Printhead-2/LConn5
  Spherical9/RConn1 -- Printhead-2/LConn4
  Spherical8/RConn1 -- Printhead-2/LConn3
  Printer Arms-8/RConn1 -- Spherical10/LConn1
  Printer Arms-7/RConn1 -- Spherical9/LConn1
  Printer Arms-3/RConn1 -- Spherical6/LConn1
  Printer Arms-4/RConn1 -- Spherical7/LConn1
  Printer Arms-5/RConn1 -- Spherical8/LConn1
  Spherical7/RConn1 -- Printhead-2/LConn2
  Spherical6/RConn1 -- Printhead-2/LConn1
  Printhead-2/RConn1 -- Body Sensor/LConn1
